simulink model "MMP2_Filter_15Hz_1kHz"  (R2016b)
settings: Solver=VariableStepAuto  StartTime=0.0  StopTime=10.0  RelTol=1e-3
settings Model: Creator=LEC3BUE  LastModifiedBy=OSS2SI
settings OptimizationCC: DefaultParameterBehavior=Inlined  UseDivisionForNetSlopeComputation=on  UseFloatMulNetSlope=on  InlineInvariantSignals=on  PassReuseOutputArgsAs=Individual arguments  ZeroExternalMemoryAtStartup=off  ZeroInternalMemoryAtStartup=off  NoFixptDivByZeroProtection=on  EfficientFloat2IntCast=on  LifeSpan=1
settings DebuggingCC: ParameterTunabilityLossMsg=error
settings RTWCC: SystemTargetFile=ert.tlc  TemplateMakefile=ert_default_tmf  Description=Embedded Coder  GenerateReport=on  IncludeHyperlinkInReport=on  LaunchReport=on  GenerateTraceInfo=on  GenerateTraceReport=on  GenerateTraceReportSl=on  GenerateTraceReportSf=on  GenerateTraceReportEml=on  GenerateCodeMetricsReport=on
settings CodeAppCC: ForceParamTrailComments=on  IgnoreCustomStorageClasses=off  OperatorAnnotations=on  SimulinkDataObjDesc=on  SFDataObjDesc=on  MATLABFcnDesc=on  CustomSymbolStrGlobalVar=rb_Mmp2_Fil_$N$M  CustomSymbolStrType=rb_Mmp2_Fil_$N$M  CustomSymbolStrField=rb_Mmp2_Fil_$N$M  CustomSymbolStrFcn=rb_Mmp2_Fil_$N$M$F  CustomSymbolStrMacro=Rb_Mmp2_Fil_$N$M  InsertBlockDesc=on  MATLABSourceComments=on
settings ERTTargetCC: TargetLangStandard=C99 (ISO)  GenerateSampleERTMain=on  CombineSignalStateStructs=on  SupportComplex=off  SupportContinuousTime=on  InlinedParameterPlacement=NonHierarchical  RootIOFormat=Structure reference  ERTCustomFileTemplate=example_file_process.tlc  ERTFilePackagingFormat=CompactWithDataFile

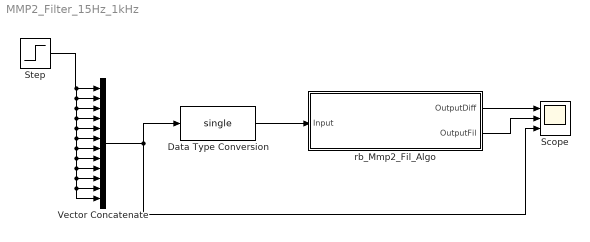
== system MMP2_Filter_15Hz_1kHz ==
  Data Type Conversion : DataTypeConversion  OutDataTypeStr=single
  Scope : Scope  NumInputPorts=3
  Step : Step  SampleTime=0
  Vector Concatenate : Concatenate  NumInputs=12
  rb_Mmp2_Fil_Algo : Subsystem
  wires:
  Data Type Conversion/1 -> rb_Mmp2_Fil_Algo/1(Input)
  rb_Mmp2_Fil_Algo/1(OutputDiff) -> Scope/1
  rb_Mmp2_Fil_Algo/2(OutputFil) -> Scope/2
  Vector Concatenate/1 -> Data Type Conversion/1, Scope/3
  Step/1 -> Vector Concatenate/12, Vector Concatenate/11, Vector Concatenate/10, Vector Concatenate/9, Vector Concatenate/8, Vector Concatenate/7, Vector Concatenate/6, Vector Concatenate/5, Vector Concatenate/4, Vector Concatenate/3, Vector Concatenate/2, Vector Concatenate/1

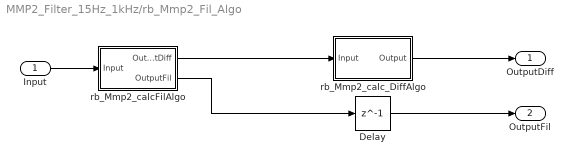
== system MMP2_Filter_15Hz_1kHz/rb_Mmp2_Fil_Algo ==
  Input : Inport
  Delay : Delay  DelayLength=1
  "rb_Mmp2_calcFilAlgo " : Subsystem  Tag=FilterWizardSubSystem
  rb_Mmp2_calc_DiffAlgo : Subsystem  Tag=FilterWizardSubSystem
      settings: ErrorFcn=dspFilterRealizedInBasicElemsAlgLoopErrFcnCallback
  OutputDiff : Outport
  OutputFil : Outport  Port=2
  wires:
  "rb_Mmp2_calcFilAlgo "/1(OutputDiff) -> rb_Mmp2_calc_DiffAlgo/1(Input)
  Input/1 -> "rb_Mmp2_calcFilAlgo "/1(Input)
  "rb_Mmp2_calcFilAlgo "/2(OutputFil) -> Delay/1
  rb_Mmp2_calc_DiffAlgo/1(Output) -> OutputDiff/1
  Delay/1 -> OutputFil/1

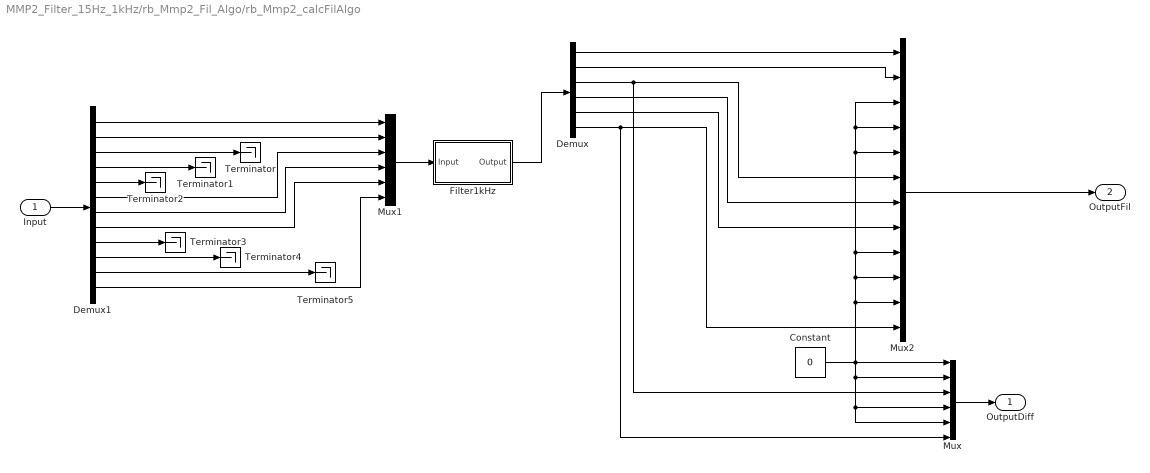
== system MMP2_Filter_15Hz_1kHz/rb_Mmp2_Fil_Algo/rb_Mmp2_calcFilAlgo  ==
  Input : Inport
  Constant : Constant  Value=0  OutDataTypeStr=single
  Demux : Demux  Outputs=6
  Demux1 : Demux  Outputs=12
  Filter1kHz : Subsystem  Tag=FilterWizardSubSystem
      settings: ErrorFcn=dspFilterRealizedInBasicElemsAlgLoopErrFcnCallback
  Mux : Mux  Inputs=6
  Mux1 : Mux  Inputs=6
  Mux2 : Mux  Inputs=12
  Terminator{,1..5} (6 alike) : Terminator
  OutputDiff : Outport
  OutputFil : Outport  Port=2
  wires:
  Mux/1 -> OutputDiff/1
  Filter1kHz/1(Output) -> Demux/1
  Demux1/1 -> Mux1/1
  Demux1/2 -> Mux1/2
  Mux1/1 -> Filter1kHz/1(Input)
  Input/1 -> Demux1/1
  Mux2/1 -> OutputFil/1
  Demux1/6 -> Mux1/3
  Demux1/7 -> Mux1/4
  Demux1/8 -> Mux1/5
  Demux1/12 -> Mux1/6
  Demux1/3 -> Terminator/1
  Demux1/4 -> Terminator1/1
  Demux1/5 -> Terminator2/1
  Demux1/9 -> Terminator3/1
  Demux1/10 -> Terminator4/1
  Demux1/11 -> Terminator5/1
  Constant/1 -> Mux/5, Mux/4, Mux/2, Mux/1, Mux2/5, Mux2/4, Mux2/3, Mux2/9, Mux2/10, Mux2/11
  Demux/1 -> Mux2/1
  Demux/2 -> Mux2/2
  Demux/3 -> Mux/3, Mux2/6
  Demux/4 -> Mux2/7
  Demux/5 -> Mux2/8
  Demux/6 -> Mux/6, Mux2/12

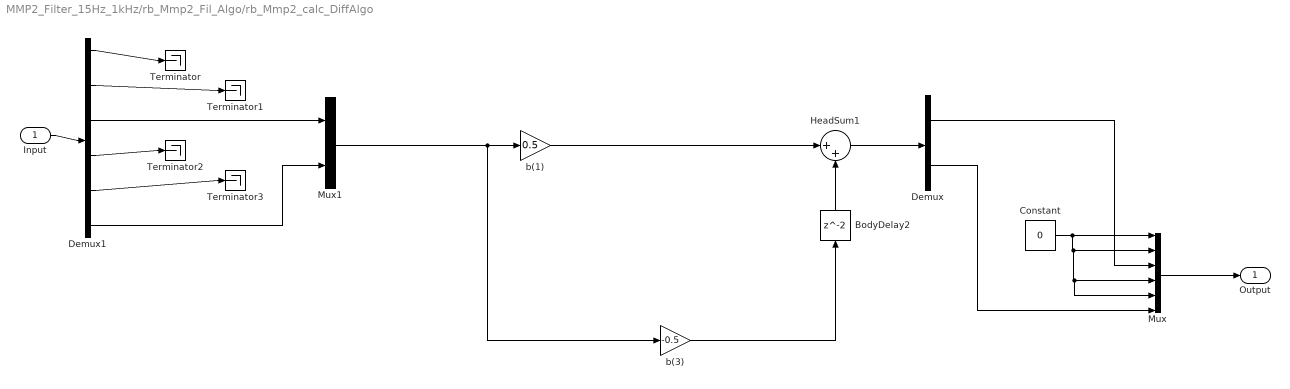
== system MMP2_Filter_15Hz_1kHz/rb_Mmp2_Fil_Algo/rb_Mmp2_calc_DiffAlgo ==
  Input : Inport
  BodyDelay2 : Delay  InitialCondition=0
  Constant : Constant  Value=0  OutDataTypeStr=single
  Demux : Demux  Outputs=2
  Demux1 : Demux  Outputs=6
  HeadSum1 : Sum  Inputs=|++  RndMeth=Nearest  SaturateOnIntegerOverflow=on  OutDataTypeStr=Inherit: Same as first input
  Mux : Mux  Inputs=6
  Mux1 : Mux  Inputs=2
  Terminator{,1..3} (4 alike) : Terminator
  b(1) : Gain  Gain=0.5  ParamDataTypeStr=single  RndMeth=Nearest  SaturateOnIntegerOverflow=on  OutDataTypeStr=Inherit: Same as input
  b(3) : Gain  Gain=-0.5  ParamDataTypeStr=single  RndMeth=Nearest  SaturateOnIntegerOverflow=on  OutDataTypeStr=Inherit: Same as input
  Output : Outport
  wires:
  b(1)/1 -> HeadSum1/1
  HeadSum1/1 -> Demux/1
  BodyDelay2/1 -> HeadSum1/2
  b(3)/1 -> BodyDelay2/1
  Input/1 -> Demux1/1
  Demux1/1 -> Terminator/1
  Demux1/2 -> Terminator1/1
  Demux1/4 -> Terminator2/1
  Demux1/5 -> Terminator3/1
  Demux1/3 -> Mux1/1
  Demux1/6 -> Mux1/2
  Mux1/1 -> b(3)/1, b(1)/1
  Constant/1 -> Mux/5, Mux/4, Mux/2, Mux/1
  Mux/1 -> Output/1
  Demux/1 -> Mux/3
  Demux/2 -> Mux/6

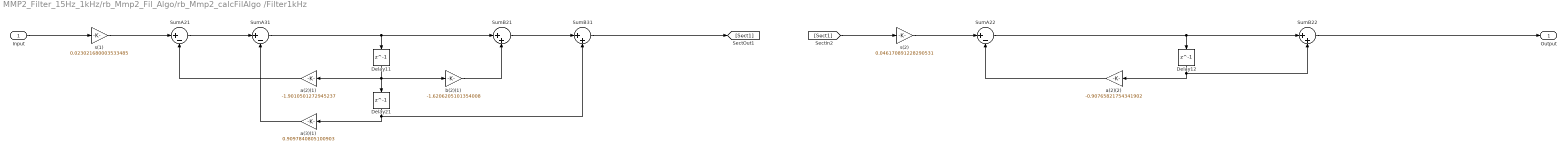
== system MMP2_Filter_15Hz_1kHz/rb_Mmp2_Fil_Algo/rb_Mmp2_calcFilAlgo /Filter1kHz ==
  Input : Inport
  Delay11 : Delay  DelayLength=1  InitialCondition=0
  Delay12 : Delay  DelayLength=1  InitialCondition=0
  Delay21 : Delay  DelayLength=1  InitialCondition=0
  SumA21 : Sum  Inputs=|+-  RndMeth=Nearest  SaturateOnIntegerOverflow=on  OutDataTypeStr=Inherit: Same as first input
  SumA22 : Sum  Inputs=|+-  RndMeth=Nearest  SaturateOnIntegerOverflow=on  OutDataTypeStr=Inherit: Same as first input
  SumA31 : Sum  Inputs=|+-  RndMeth=Nearest  SaturateOnIntegerOverflow=on  OutDataTypeStr=Inherit: Same as first input
  SumB21 : Sum  Inputs=|++  RndMeth=Nearest  SaturateOnIntegerOverflow=on  OutDataTypeStr=Inherit: Same as first input
  SumB22 : Sum  Inputs=|++  RndMeth=Nearest  SaturateOnIntegerOverflow=on  OutDataTypeStr=Inherit: Same as first input
  SumB31 : Sum  Inputs=|++  RndMeth=Nearest  SaturateOnIntegerOverflow=on  OutDataTypeStr=Inherit: Same as first input
  a(2)(1) : Gain  Gain=-1.9010501272945237  ParamDataTypeStr=double  RndMeth=Nearest  SaturateOnIntegerOverflow=on  OutDataTypeStr=Inherit: Same as input
  a(2)(2) : Gain  Gain=-0.90765821754341902  ParamDataTypeStr=double  RndMeth=Nearest  SaturateOnIntegerOverflow=on  OutDataTypeStr=Inherit: Same as input
  a(3)(1) : Gain  Gain=0.9097840805100903  ParamDataTypeStr=double  RndMeth=Nearest  SaturateOnIntegerOverflow=on  OutDataTypeStr=Inherit: Same as input
  b(2)(1) : Gain  Gain=-1.6206205101354008  ParamDataTypeStr=double  RndMeth=Nearest  SaturateOnIntegerOverflow=on  OutDataTypeStr=Inherit: Same as input
  s(1) : Gain  Gain=0.023021680003533485  ParamDataTypeStr=double  RndMeth=Nearest  SaturateOnIntegerOverflow=on  OutDataTypeStr=Inherit: Same as input
  s(2) : Gain  Gain=0.046170891228290531  ParamDataTypeStr=double  RndMeth=Nearest  SaturateOnIntegerOverflow=on  OutDataTypeStr=Inherit: Same as input
  Output : Outport
  wires:
  Input/1 -> s(1)/1
  s(1)/1 -> SumA21/1
  SumA21/1 -> SumA31/1
  SumA31/1 -> SumB21/1, Delay11/1
  SumB21/1 -> SumB31/1
  SumB31/1 -> [Sect1]
  a(2)(1)/1 -> SumA21/2
  Delay11/1 -> a(2)(1)/1, b(2)(1)/1, Delay21/1
  b(2)(1)/1 -> SumB21/2
  a(3)(1)/1 -> SumA31/2
  Delay21/1 -> a(3)(1)/1, SumB31/2
  [Sect1] -> s(2)/1
  s(2)/1 -> SumA22/1
  SumA22/1 -> SumB22/1, Delay12/1
  SumB22/1 -> Output/1
  a(2)(2)/1 -> SumA22/2
  Delay12/1 -> a(2)(2)/1, SumB22/2
